simulink model "sampleModel7126_pp_difftest"  (R2018a)
settings: Solver=VariableStepAuto  StartTime=0.0  StopTime=10.0  RelTol=1e-3
undefined symbols (not defined in the file or in its folder): DiscIntNeverNeededParam
libraries: simulink x367
(part 5 of 8)

== system sampleModel7126_pp_difftest/cfblk293 ==
  cfblk1 : Inport
  cfblk9 : Inport  Port=2
  Action Port : ActionPort  ActionType=then
  cfblk{6,10..13} (5 alike) : Delay
  cfblk3 : simulink/Continuous/PID Controller (2DOF)  Controller=PID  TimeDomain=Discrete-time  SampleTime=-1  IntegratorMethod=Forward Euler  FilterMethod=Forward Euler  Form=Parallel  UseFilter=on  ControllerParametersSource=internal  P=1  I=1  D=0  N=100  b=1  c=1  InitialConditionSource=internal  InitialConditionForIntegrator=0  InitialConditionForFilter=0  ExternalReset=none  LimitOutput=off  UpperSaturationLimit=inf  LowerSaturationLimit=-inf  LinearizeAsGain=off  AntiWindupMode=none  Kb=1  TrackingMode=off  Kt=1  PParamMin=[]  PParamMax=[]  IParamMin=[]  IParamMax=[]  DParamMin=[]  DParamMax=[]  NParamMin=[]  NParamMax=[]  bParamMin=[]  bParamMax=[]  cParamMin=[]  cParamMax=[]  KbParamMin=[]  KbParamMax=[]  KtParamMin=[]  KtParamMax=[]  POutMin=[]  POutMax=[]  IOutMin=[]  IOutMax=[]  DOutMin=[]  DOutMax=[]  NOutMin=[]  NOutMax=[]  bOutMin=[]  bOutMax=[]  cOutMin=[]  cOutMax=[]  KbOutMin=[]  KbOutMax=[]  KtOutMin=[]  KtOutMax=[]  IntegratorOutMin=[]  IntegratorOutMax=[]  FilterOutMin=[]  FilterOutMax=[]  SumOutMin=[]  SumOutMax=[]  Sum1OutMin=[]  Sum1OutMax=[]  Sum2OutMin=[]  Sum2OutMax=[]  Sum3OutMin=[]  Sum3OutMax=[]  SumI1OutMin=[]  SumI1OutMax=[]  SumI2OutMin=[]  SumI2OutMax=[]  SumI3OutMin=[]  SumI3OutMax=[]  SumDOutMin=[]  SumDOutMax=[]  SaturationOutMin=[]  SaturationOutMax=[]  IntegratorContinuousStateAttributes=''  IntegratorStateMustResolveToSignalObject=off  IntegratorRTWStateStorageClass=Auto  FilterContinuousStateAttributes=''  FilterStateMustResolveToSignalObject=off  FilterRTWStateStorageClass=Auto  DifferentiatorICPrevScaledInput=0  DifferentiatorOutMin=[]  DifferentiatorOutMax=[]  FilterDiffOutCoefMin=[]  FilterDiffOutCoefMax=[]  SumDenOutMin=[]  SumDenOutMax=[]  SumNumOutMin=[]  SumNumOutMax=[]  ReciprocalOutMin=[]  ReciprocalOutMax=[]  DivideOutMin=[]  DivideOutMax=[]  TunerSelectOption=Transfer Function Based (PID Tuner App)
  cfblk4 : Delay  ShowEnablePort=on
      settings: InputPortMap=u0,e6
  cfblk5 : Delay  ShowEnablePort=on
      settings: InputPortMap=u0,e6
  cfblk7 : simulink/Continuous/PID Controller (2DOF)  Controller=PID  TimeDomain=Discrete-time  SampleTime=-1  IntegratorMethod=Forward Euler  FilterMethod=Forward Euler  Form=Parallel  UseFilter=on  ControllerParametersSource=internal  P=1  I=1  D=0  N=100  b=1  c=1  InitialConditionSource=internal  InitialConditionForIntegrator=0  InitialConditionForFilter=0  ExternalReset=none  LimitOutput=off  UpperSaturationLimit=inf  LowerSaturationLimit=-inf  LinearizeAsGain=off  AntiWindupMode=none  Kb=1  TrackingMode=off  Kt=1  PParamMin=[]  PParamMax=[]  IParamMin=[]  IParamMax=[]  DParamMin=[]  DParamMax=[]  NParamMin=[]  NParamMax=[]  bParamMin=[]  bParamMax=[]  cParamMin=[]  cParamMax=[]  KbParamMin=[]  KbParamMax=[]  KtParamMin=[]  KtParamMax=[]  POutMin=[]  POutMax=[]  IOutMin=[]  IOutMax=[]  DOutMin=[]  DOutMax=[]  NOutMin=[]  NOutMax=[]  bOutMin=[]  bOutMax=[]  cOutMin=[]  cOutMax=[]  KbOutMin=[]  KbOutMax=[]  KtOutMin=[]  KtOutMax=[]  IntegratorOutMin=[]  IntegratorOutMax=[]  FilterOutMin=[]  FilterOutMax=[]  SumOutMin=[]  SumOutMax=[]  Sum1OutMin=[]  Sum1OutMax=[]  Sum2OutMin=[]  Sum2OutMax=[]  Sum3OutMin=[]  Sum3OutMax=[]  SumI1OutMin=[]  SumI1OutMax=[]  SumI2OutMin=[]  SumI2OutMax=[]  SumI3OutMin=[]  SumI3OutMax=[]  SumDOutMin=[]  SumDOutMax=[]  SaturationOutMin=[]  SaturationOutMax=[]  IntegratorContinuousStateAttributes=''  IntegratorStateMustResolveToSignalObject=off  IntegratorRTWStateStorageClass=Auto  FilterContinuousStateAttributes=''  FilterStateMustResolveToSignalObject=off  FilterRTWStateStorageClass=Auto  DifferentiatorICPrevScaledInput=0  DifferentiatorOutMin=[]  DifferentiatorOutMax=[]  FilterDiffOutCoefMin=[]  FilterDiffOutCoefMax=[]  SumDenOutMin=[]  SumDenOutMax=[]  SumNumOutMin=[]  SumNumOutMax=[]  ReciprocalOutMin=[]  ReciprocalOutMax=[]  DivideOutMin=[]  DivideOutMax=[]  TunerSelectOption=Transfer Function Based (PID Tuner App)
  cfblk8 : simulink/Discrete/Transfer Fcn First Order  PoleZ=0.95  ICPrevOutput=0.0  DoSatur=off
      settings: SourceProductName=Simulink
  cyemi_{1188..1201} (14 alike) : DataTypeConversion  OutDataTypeStr=double
  cfblk2 : Outport
  wires:
  cfblk7/1 -> cyemi_1189/1, cyemi_1190/1, cyemi_1191/1
  cfblk1/1 -> cfblk2/1
  cfblk8/1 -> cyemi_1188/1, cyemi_1200/1
  cyemi_1188/1 -> cfblk10/1
  cyemi_1189/1 -> cfblk11/1
  cyemi_1190/1 -> cfblk12/1
  cyemi_1191/1 -> cfblk13/1
  cyemi_1192/1 -> cfblk3/1
  cfblk10/1 -> cyemi_1192/1
  cyemi_1193/1 -> cfblk3/2
  cfblk13/1 -> cyemi_1193/1
  cyemi_1194/1 -> cfblk4/1
  cfblk5/1 -> cyemi_1194/1
  cyemi_1195/1 -> cfblk4/2
  cfblk12/1 -> cyemi_1195/1
  cyemi_1196/1 -> cfblk5/1
  cfblk11/1 -> cyemi_1196/1
  cyemi_1197/1 -> cfblk5/2
  cfblk3/1 -> cyemi_1197/1
  cyemi_1198/1 -> cfblk6/1
  cfblk4/1 -> cyemi_1198/1
  cyemi_1199/1 -> cfblk7/1
  cfblk9/1 -> cyemi_1199/1
  cyemi_1200/1 -> cfblk7/2
  cyemi_1201/1 -> cfblk8/1
  cfblk6/1 -> cyemi_1201/1

== system sampleModel7126_pp_difftest/cfblk294 ==
  cfblk1 : Inport
  cfblk9 : Inport  Port=2
  cfblk10 : Inport  Port=3
  Action Port : ActionPort  ActionType=else
  cfblk11 : Delay
  cfblk12 : Delay
  cfblk3 : Delay  DelayLengthSource=Input port
      settings: InputPortMap=u0,p1
  cfblk4 : Delay  DelayLengthSource=Input port
      settings: InputPortMap=u0,p1
  cfblk5 : simulink/Discrete/Tapped Delay  vinit=0.0  samptime=-1  NumDelays=1  DelayOrder=Oldest  includeCurrent=off
  cfblk6 : Delay  DelayLengthSource=Input port
      settings: InputPortMap=u0,p1
  cfblk7 : Delay
  cfblk8 : simulink/Discrete/Transfer Fcn First Order  PoleZ=0.95  ICPrevOutput=0.0  DoSatur=off
      settings: SourceProductName=Simulink
  cyemi_{1205..1215} (11 alike) : DataTypeConversion  OutDataTypeStr=double
  cfblk2 : Outport
  wires:
  cfblk9/1 -> cfblk2/1
  cfblk7/1 -> cyemi_1209/1, cyemi_1211/1
  cyemi_1205/1 -> cfblk11/1
  cfblk8/1 -> cyemi_1205/1
  cyemi_1206/1 -> cfblk12/1
  cfblk6/1 -> cyemi_1206/1
  cyemi_1207/1 -> cfblk3/1
  cfblk11/1 -> cyemi_1207/1
  cyemi_1208/1 -> cfblk3/2
  cfblk1/1 -> cyemi_1208/1
  cyemi_1209/1 -> cfblk4/1
  cyemi_1210/1 -> cfblk4/2
  cfblk12/1 -> cyemi_1210/1
  cyemi_1211/1 -> cfblk5/1
  cyemi_1212/1 -> cfblk6/1
  cfblk5/1 -> cyemi_1212/1
  cyemi_1213/1 -> cfblk6/2
  cfblk4/1 -> cyemi_1213/1
  cyemi_1214/1 -> cfblk7/1
  cfblk10/1 -> cyemi_1214/1
  cyemi_1215/1 -> cfblk8/1
  cfblk3/1 -> cyemi_1215/1

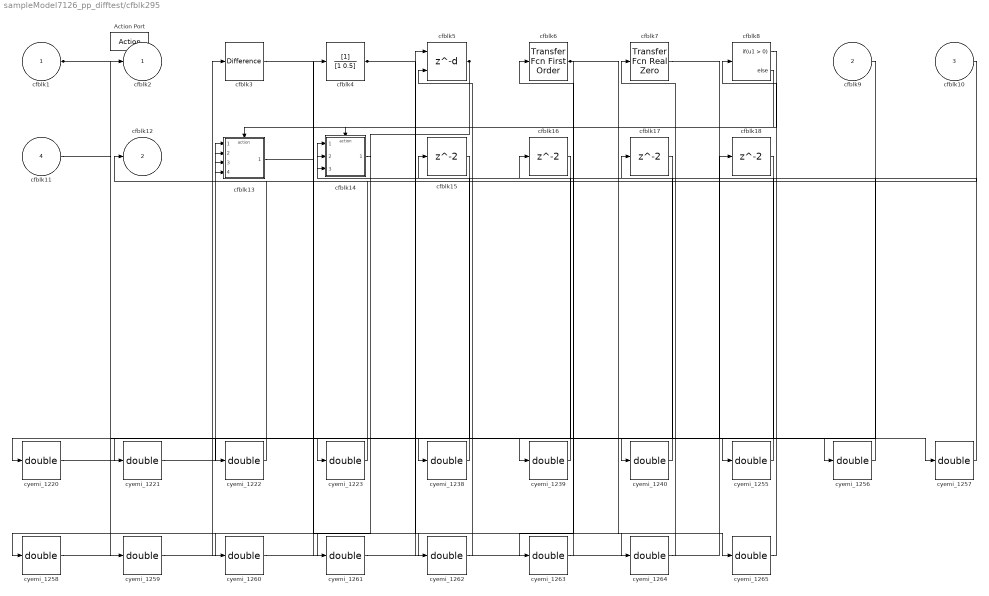
== system sampleModel7126_pp_difftest/cfblk295 ==
  cfblk1 : Inport
  cfblk9 : Inport  Port=2
  cfblk10 : Inport  Port=3
  cfblk11 : Inport  Port=4
  Action Port : ActionPort  ActionType=then
  cfblk13 : Subsystem  TreatAsAtomicUnit=on
  cfblk14 : Subsystem  TreatAsAtomicUnit=on
  cfblk{15..18} (4 alike) : Delay
  cfblk3 : simulink/Discrete/Difference  ICPrevInput=0.0  OutMin=[]  OutMax=[]  OutDataTypeStr=double  OutputDataTypeScalingMode=double  OutDataType=fixdt(1, 16)  OutScaling=2^-10  DoSatur=off
  cfblk4 : DiscreteFilter
  cfblk5 : Delay  DelayLengthSource=Input port
      settings: InputPortMap=u0,p1
  cfblk6 : simulink/Discrete/Transfer Fcn First Order  PoleZ=0.95  ICPrevOutput=0.0  DoSatur=off
      settings: SourceProductName=Simulink
  cfblk7 : simulink/Discrete/Transfer Fcn Real Zero  ZeroZ=0.75  ICPrevInput=0.0  DoSatur=off
      settings: SourceProductName=Simulink  SourceProductBaseCode=SL
  cfblk8 : If  SampleTime=1
  cyemi_{1220..1223,1238..1240,1255..1265} (18 alike) : DataTypeConversion  OutDataTypeStr=double
  cfblk2 : Outport
  cfblk12 : Outport  Port=2
  wires:
  cfblk4/1 -> cyemi_1255/1, cyemi_1264/1
  cfblk5/1 -> cyemi_1258/1, cyemi_1260/1
  cfblk10/1 -> cfblk12/1
  cfblk1/1 -> cfblk2/1, cyemi_1223/1, cyemi_1240/1
  cfblk6/1 -> cyemi_1239/1, cyemi_1265/1
  cfblk8/1 -> cfblk13/Action
  cfblk8/2 -> cfblk14/Action
  cyemi_1220/1 -> cfblk13/1(cfblk1)
  cfblk15/1 -> cyemi_1220/1
  cyemi_1221/1 -> cfblk13/2(cfblk15)
  cfblk17/1 -> cyemi_1221/1
  cyemi_1222/1 -> cfblk13/3(cfblk16)
  cfblk18/1 -> cyemi_1222/1
  cyemi_1223/1 -> cfblk13/4(cfblk17)
  cyemi_1238/1 -> cfblk14/1(cfblk1)
  cfblk16/1 -> cyemi_1238/1
  cyemi_1239/1 -> cfblk14/2(cfblk14)
  cyemi_1240/1 -> cfblk14/3(cfblk15)
  cyemi_1255/1 -> cfblk15/1
  cyemi_1256/1 -> cfblk16/1
  cfblk13/1(cfblk2) -> cyemi_1256/1
  cyemi_1257/1 -> cfblk17/1
  cfblk7/1 -> cyemi_1257/1
  cyemi_1258/1 -> cfblk18/1
  cyemi_1259/1 -> cfblk3/1
  cfblk11/1 -> cyemi_1259/1
  cyemi_1260/1 -> cfblk4/1
  cyemi_1261/1 -> cfblk5/1
  cfblk14/1(cfblk2) -> cyemi_1261/1
  cyemi_1262/1 -> cfblk5/2
  cfblk3/1 -> cyemi_1262/1
  cyemi_1263/1 -> cfblk6/1
  cfblk9/1 -> cyemi_1263/1
  cyemi_1264/1 -> cfblk7/1
  cyemi_1265/1 -> cfblk8/1

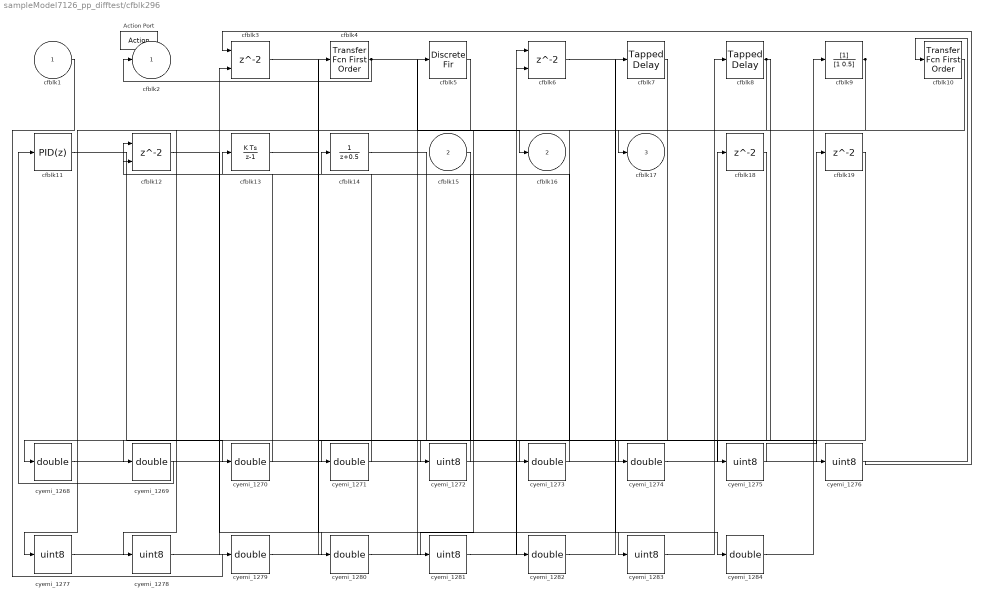
== system sampleModel7126_pp_difftest/cfblk296 ==
  cfblk1 : Inport
  cfblk15 : Inport  Port=2
  Action Port : ActionPort  ActionType=else
  cfblk10 : simulink/Discrete/Transfer Fcn First Order  PoleZ=0.95  ICPrevOutput=0.0  DoSatur=off
      settings: SourceProductName=Simulink
  cfblk11 : simulink/Continuous/PID Controller  Controller=PID  TimeDomain=Discrete-time  SampleTime=-1  IntegratorMethod=Forward Euler  FilterMethod=Forward Euler  Form=Parallel  UseFilter=on  ControllerParametersSource=internal  P=1  I=1  D=0  N=100  InitialConditionSource=internal  InitialConditionForIntegrator=0  InitialConditionForFilter=0  ExternalReset=none  LimitOutput=off  UpperSaturationLimit=inf  LowerSaturationLimit=-inf  LinearizeAsGain=off  AntiWindupMode=none  Kb=1  TrackingMode=off  Kt=1  PParamMin=[]  PParamMax=[]  IParamMin=[]  IParamMax=[]  DParamMin=[]  DParamMax=[]  NParamMin=[]  NParamMax=[]  KbParamMin=[]  KbParamMax=[]  KtParamMin=[]  KtParamMax=[]  POutMin=[]  POutMax=[]  IOutMin=[]  IOutMax=[]  DOutMin=[]  DOutMax=[]  NOutMin=[]  NOutMax=[]  KbOutMin=[]  KbOutMax=[]  KtOutMin=[]  KtOutMax=[]  IntegratorOutMin=[]  IntegratorOutMax=[]  FilterOutMin=[]  FilterOutMax=[]  SumOutMin=[]  SumOutMax=[]  SumI1OutMin=[]  SumI1OutMax=[]  SumI2OutMin=[]  SumI2OutMax=[]  SumI3OutMin=[]  SumI3OutMax=[]  SumDOutMin=[]  SumDOutMax=[]  SaturationOutMin=[]  SaturationOutMax=[]  IntegratorContinuousStateAttributes=''  IntegratorStateMustResolveToSignalObject=off  IntegratorRTWStateStorageClass=Auto  FilterContinuousStateAttributes=''  FilterStateMustResolveToSignalObject=off  FilterRTWStateStorageClass=Auto  DifferentiatorICPrevScaledInput=0  DifferentiatorOutMin=[]  DifferentiatorOutMax=[]  FilterDiffOutCoefMin=[]  FilterDiffOutCoefMax=[]  SumDenOutMin=[]  SumDenOutMax=[]  SumNumOutMin=[]  SumNumOutMax=[]  ReciprocalOutMin=[]  ReciprocalOutMax=[]  DivideOutMin=[]  DivideOutMax=[]  TunerSelectOption=Transfer Function Based (PID Tuner App)
  cfblk12 : Delay  ShowEnablePort=on
      settings: InputPortMap=u0,e6
  cfblk13 : DiscreteIntegrator  SampleTime=-1  OutDataTypeStr=uint8  ICPrevOutput=DiscIntNeverNeededParam  ICPrevScaledInput=DiscIntNeverNeededParam
  cfblk14 : DiscreteTransferFcn
  cfblk18 : Delay
  cfblk19 : Delay
  cfblk3 : Delay  ShowEnablePort=on
      settings: InputPortMap=u0,e6
  cfblk4 : simulink/Discrete/Transfer Fcn First Order  PoleZ=0.95  ICPrevOutput=0.0  DoSatur=off
      settings: SourceProductName=Simulink
  cfblk5 : DiscreteFir
  cfblk6 : Delay  ShowEnablePort=on
      settings: InputPortMap=u0,e6
  cfblk7 : simulink/Discrete/Tapped Delay  vinit=0.0  samptime=-1  NumDelays=1  DelayOrder=Oldest  includeCurrent=off
  cfblk8 : simulink/Discrete/Tapped Delay  vinit=0.0  samptime=-1  NumDelays=1  DelayOrder=Oldest  includeCurrent=off
  cfblk9 : DiscreteFilter
  cyemi_{1268..1271,1273..1274,1279..1280,1282,1284} (10 alike) : DataTypeConversion  OutDataTypeStr=double
  cyemi_{1272,1275..1278,1281,1283} (7 alike) : DataTypeConversion  OutDataTypeStr=uint8
  cfblk2 : Outport
  cfblk16 : Outport  Port=2
  cfblk17 : Outport  Port=3
  wires:
  cfblk10/1 -> cfblk17/1
  cfblk4/1 -> cfblk2/1, cfblk16/1
  cfblk8/1 -> cyemi_1275/1, cyemi_1278/1, cyemi_1281/1
  cfblk9/1 -> cyemi_1268/1, cyemi_1273/1
  cyemi_1268/1 -> cfblk10/1
  cyemi_1269/1 -> cfblk11/1
  cfblk5/1 -> cyemi_1269/1
  cyemi_1270/1 -> cfblk12/1
  cfblk11/1 -> cyemi_1270/1
  cyemi_1271/1 -> cfblk12/2
  cfblk18/1 -> cyemi_1271/1
  cyemi_1272/1 -> cfblk13/1
  cfblk15/1 -> cyemi_1272/1
  cyemi_1273/1 -> cfblk14/1
  cyemi_1274/1 -> cfblk18/1
  cfblk7/1 -> cyemi_1274/1
  cyemi_1275/1 -> cfblk19/1
  cyemi_1276/1 -> cfblk3/1
  cfblk13/1 -> cyemi_1276/1
  cyemi_1277/1 -> cfblk3/2
  cfblk19/1 -> cyemi_1277/1
  cyemi_1278/1 -> cfblk4/1
  cyemi_1279/1 -> cfblk5/1
  cfblk1/1 -> cyemi_1279/1
  cyemi_1280/1 -> cfblk6/1
  cfblk12/1 -> cyemi_1280/1
  cyemi_1281/1 -> cfblk6/2
  cyemi_1282/1 -> cfblk7/1
  cfblk14/1 -> cyemi_1282/1
  cyemi_1283/1 -> cfblk8/1
  cfblk3/1 -> cyemi_1283/1
  cyemi_1284/1 -> cfblk9/1
  cfblk6/1 -> cyemi_1284/1

== system sampleModel7126_pp_difftest/cfblk297 ==
  cfblk1 : Inport
  cfblk8 : Inport  Port=2
  cfblk9 : Inport  Port=3
  Action Port : ActionPort  ActionType=then
  cfblk11 : Delay
  cfblk3 : DiscreteFilter
  cfblk4 : simulink/Discrete/Tapped Delay  vinit=0.0  samptime=-1  NumDelays=1  DelayOrder=Oldest  includeCurrent=off
  cfblk5 : simulink/Continuous/PID Controller  Controller=PID  TimeDomain=Discrete-time  SampleTime=-1  IntegratorMethod=Forward Euler  FilterMethod=Forward Euler  Form=Parallel  UseFilter=on  ControllerParametersSource=internal  P=1  I=1  D=0  N=100  InitialConditionSource=internal  InitialConditionForIntegrator=0  InitialConditionForFilter=0  ExternalReset=none  LimitOutput=off  UpperSaturationLimit=inf  LowerSaturationLimit=-inf  LinearizeAsGain=off  AntiWindupMode=none  Kb=1  TrackingMode=off  Kt=1  PParamMin=[]  PParamMax=[]  IParamMin=[]  IParamMax=[]  DParamMin=[]  DParamMax=[]  NParamMin=[]  NParamMax=[]  KbParamMin=[]  KbParamMax=[]  KtParamMin=[]  KtParamMax=[]  POutMin=[]  POutMax=[]  IOutMin=[]  IOutMax=[]  DOutMin=[]  DOutMax=[]  NOutMin=[]  NOutMax=[]  KbOutMin=[]  KbOutMax=[]  KtOutMin=[]  KtOutMax=[]  IntegratorOutMin=[]  IntegratorOutMax=[]  FilterOutMin=[]  FilterOutMax=[]  SumOutMin=[]  SumOutMax=[]  SumI1OutMin=[]  SumI1OutMax=[]  SumI2OutMin=[]  SumI2OutMax=[]  SumI3OutMin=[]  SumI3OutMax=[]  SumDOutMin=[]  SumDOutMax=[]  SaturationOutMin=[]  SaturationOutMax=[]  IntegratorContinuousStateAttributes=''  IntegratorStateMustResolveToSignalObject=off  IntegratorRTWStateStorageClass=Auto  FilterContinuousStateAttributes=''  FilterStateMustResolveToSignalObject=off  FilterRTWStateStorageClass=Auto  DifferentiatorICPrevScaledInput=0  DifferentiatorOutMin=[]  DifferentiatorOutMax=[]  FilterDiffOutCoefMin=[]  FilterDiffOutCoefMax=[]  SumDenOutMin=[]  SumDenOutMax=[]  SumNumOutMin=[]  SumNumOutMax=[]  ReciprocalOutMin=[]  ReciprocalOutMax=[]  DivideOutMin=[]  DivideOutMax=[]  TunerSelectOption=Transfer Function Based (PID Tuner App)
  cfblk6 : simulink/Discrete/Difference  ICPrevInput=0.0  OutMin=[]  OutMax=[]  OutDataTypeStr=double  OutputDataTypeScalingMode=double  OutDataType=fixdt(1, 16)  OutScaling=2^-10  DoSatur=off
  cfblk7 : simulink/Continuous/PID Controller (2DOF)  Controller=PID  TimeDomain=Discrete-time  SampleTime=-1  IntegratorMethod=Forward Euler  FilterMethod=Forward Euler  Form=Parallel  UseFilter=on  ControllerParametersSource=internal  P=1  I=1  D=0  N=100  b=1  c=1  InitialConditionSource=internal  InitialConditionForIntegrator=0  InitialConditionForFilter=0  ExternalReset=none  LimitOutput=off  UpperSaturationLimit=inf  LowerSaturationLimit=-inf  LinearizeAsGain=off  AntiWindupMode=none  Kb=1  TrackingMode=off  Kt=1  PParamMin=[]  PParamMax=[]  IParamMin=[]  IParamMax=[]  DParamMin=[]  DParamMax=[]  NParamMin=[]  NParamMax=[]  bParamMin=[]  bParamMax=[]  cParamMin=[]  cParamMax=[]  KbParamMin=[]  KbParamMax=[]  KtParamMin=[]  KtParamMax=[]  POutMin=[]  POutMax=[]  IOutMin=[]  IOutMax=[]  DOutMin=[]  DOutMax=[]  NOutMin=[]  NOutMax=[]  bOutMin=[]  bOutMax=[]  cOutMin=[]  cOutMax=[]  KbOutMin=[]  KbOutMax=[]  KtOutMin=[]  KtOutMax=[]  IntegratorOutMin=[]  IntegratorOutMax=[]  FilterOutMin=[]  FilterOutMax=[]  SumOutMin=[]  SumOutMax=[]  Sum1OutMin=[]  Sum1OutMax=[]  Sum2OutMin=[]  Sum2OutMax=[]  Sum3OutMin=[]  Sum3OutMax=[]  SumI1OutMin=[]  SumI1OutMax=[]  SumI2OutMin=[]  SumI2OutMax=[]  SumI3OutMin=[]  SumI3OutMax=[]  SumDOutMin=[]  SumDOutMax=[]  SaturationOutMin=[]  SaturationOutMax=[]  IntegratorContinuousStateAttributes=''  IntegratorStateMustResolveToSignalObject=off  IntegratorRTWStateStorageClass=Auto  FilterContinuousStateAttributes=''  FilterStateMustResolveToSignalObject=off  FilterRTWStateStorageClass=Auto  DifferentiatorICPrevScaledInput=0  DifferentiatorOutMin=[]  DifferentiatorOutMax=[]  FilterDiffOutCoefMin=[]  FilterDiffOutCoefMax=[]  SumDenOutMin=[]  SumDenOutMax=[]  SumNumOutMin=[]  SumNumOutMax=[]  ReciprocalOutMin=[]  ReciprocalOutMax=[]  DivideOutMin=[]  DivideOutMax=[]  TunerSelectOption=Transfer Function Based (PID Tuner App)
  cyemi_{1288..1294} (7 alike) : DataTypeConversion  OutDataTypeStr=double
  cfblk2 : Outport
  cfblk10 : Outport  Port=2
  wires:
  cfblk1/1 -> cfblk10/1
  cfblk6/1 -> cfblk2/1
  cyemi_1288/1 -> cfblk11/1
  cfblk7/1 -> cyemi_1288/1
  cyemi_1289/1 -> cfblk3/1
  cfblk11/1 -> cyemi_1289/1
  cyemi_1290/1 -> cfblk4/1
  cfblk9/1 -> cyemi_1290/1
  cyemi_1291/1 -> cfblk5/1
  cfblk8/1 -> cyemi_1291/1
  cyemi_1292/1 -> cfblk6/1
  cfblk4/1 -> cyemi_1292/1
  cyemi_1293/1 -> cfblk7/1
  cfblk5/1 -> cyemi_1293/1
  cyemi_1294/1 -> cfblk7/2
  cfblk3/1 -> cyemi_1294/1

== system sampleModel7126_pp_difftest/cfblk298 ==
  cfblk1 : Inport
  cfblk9 : Inport  Port=2
  cfblk10 : Inport  Port=3
  cfblk11 : Inport  Port=4
  Action Port : ActionPort  ActionType=else
  cfblk15 : Subsystem  TreatAsAtomicUnit=on
  cfblk16 : Subsystem  TreatAsAtomicUnit=on
  cfblk{3..4,17..19} (5 alike) : Delay
  cfblk5 : DiscreteZeroPole  Poles=[0 0.5]  Gain=1  SampleTime=-1
  cfblk6 : DiscreteZeroPole  Poles=[0 0.5]  Gain=1  SampleTime=-1
  cfblk7 : DiscreteFilter
  cfblk8 : If  SampleTime=1
  cyemi_{1299..1300,1314,1331..1339} (12 alike) : DataTypeConversion  OutDataTypeStr=double
  cfblk2 : Outport
  cfblk12 : Outport  Port=2
  cfblk13 : Outport  Port=3
  cfblk14 : Outport  Port=4
  wires:
  cfblk10/1 -> cfblk14/1
  cfblk4/1 -> cfblk2/1
  cfblk15/1(cfblk2) -> cfblk12/1
  cfblk9/1 -> cfblk13/1
  cfblk8/1 -> cfblk15/Action
  cfblk8/2 -> cfblk16/Action
  cyemi_1299/1 -> cfblk15/1(cfblk1)
  cfblk11/1 -> cyemi_1299/1, cyemi_1300/1
  cyemi_1300/1 -> cfblk15/2(cfblk14)
  cyemi_1314/1 -> cfblk16/1(cfblk1)
  cfblk7/1 -> cyemi_1314/1
  cyemi_1331/1 -> cfblk17/1
  cfblk6/1 -> cyemi_1331/1
  cyemi_1332/1 -> cfblk18/1
  cfblk16/1(cfblk2) -> cyemi_1332/1
  cyemi_1333/1 -> cfblk19/1
  cfblk15/2(cfblk15) -> cyemi_1333/1
  cyemi_1334/1 -> cfblk3/1
  cfblk17/1 -> cyemi_1334/1
  cyemi_1335/1 -> cfblk4/1
  cfblk1/1 -> cyemi_1335/1
  cyemi_1336/1 -> cfblk5/1
  cfblk18/1 -> cyemi_1336/1
  cyemi_1337/1 -> cfblk6/1
  cfblk3/1 -> cyemi_1337/1
  cyemi_1338/1 -> cfblk7/1
  cfblk5/1 -> cyemi_1338/1
  cyemi_1339/1 -> cfblk8/1
  cfblk19/1 -> cyemi_1339/1

== system sampleModel7126_pp_difftest/cfblk245/cfblk18 ==
  cfblk1 : Inport
  cfblk9 : Inport  Port=2
  Action Port : ActionPort  ActionType=then
  cfblk3 : UnitDelay  SampleTime=-1
  cfblk4 : Delay  ShowEnablePort=on
      settings: InputPortMap=u0,e6
  cfblk5 : DiscreteFilter
  cfblk6 : simulink/Discrete/Transfer Fcn Real Zero  ZeroZ=0.75  ICPrevInput=0.0  DoSatur=off
      settings: SourceProductName=Simulink  SourceProductBaseCode=SL
  cfblk7 : simulink/Discrete/Transfer Fcn Lead or Lag  PoleZ=0.95  ZeroZ=0.75  ICPrevOutput=0.0  ICPrevInput=0.0  DoSatur=off
      settings: SourceProductName=Simulink  SourceProductBaseCode=SL
  cfblk8 : Delay  DelayLengthSource=Input port
      settings: InputPortMap=u0,p1
  cyemi_{71..78} (8 alike) : DataTypeConversion  OutDataTypeStr=double
  cfblk2 : Outport
  cfblk10 : Outport  Port=2
  cfblk11 : Outport  Port=3
  wires:
  cfblk5/1 -> cfblk11/1
  cfblk3/1 -> cfblk10/1, cyemi_73/1, cyemi_74/1
  cfblk8/1 -> cfblk2/1
  cyemi_71/1 -> cfblk3/1
  cfblk7/1 -> cyemi_71/1
  cyemi_72/1 -> cfblk4/1
  cfblk6/1 -> cyemi_72/1
  cyemi_73/1 -> cfblk4/2
  cyemi_74/1 -> cfblk5/1
  cyemi_75/1 -> cfblk6/1
  cfblk9/1 -> cyemi_75/1
  cyemi_76/1 -> cfblk7/1
  cfblk1/1 -> cyemi_76/1
  cyemi_77/1 -> cfblk8/1
  cfblk4/1 -> cyemi_77/1, cyemi_78/1
  cyemi_78/1 -> cfblk8/2

== system sampleModel7126_pp_difftest/cfblk245/cfblk19 ==
  cfblk1 : Inport
  Action Port : ActionPort  ActionType=else
  cfblk10 : DiscreteZeroPole  Poles=[0 0.5]  Gain=1  SampleTime=-1
  cfblk13 : Delay
  cfblk3 : DiscreteStateSpace  SampleTime=-1
  cfblk4 : DiscreteZeroPole  Poles=[0 0.5]  Gain=1  SampleTime=-1
  cfblk5 : DiscreteZeroPole  Poles=[0 0.5]  Gain=1  SampleTime=-1
  cfblk6 : simulink/Discrete/Transfer Fcn First Order  PoleZ=0.95  ICPrevOutput=0.0  DoSatur=off
      settings: SourceProductName=Simulink
  cfblk7 : DiscreteFir
  cfblk8 : DiscreteIntegrator  SampleTime=-1  OutDataTypeStr=double  ICPrevOutput=DiscIntNeverNeededParam  ICPrevScaledInput=DiscIntNeverNeededParam
  cfblk9 : Delay  ShowEnablePort=on
      settings: InputPortMap=u0,e6
  cyemi_{80..89} (10 alike) : DataTypeConversion  OutDataTypeStr=double
  cfblk2 : Outport
  cfblk11 : Outport  Port=2
  cfblk12 : Outport  Port=3
  wires:
  cfblk8/1 -> cyemi_85/1, cyemi_88/1
  cfblk5/1 -> cfblk11/1, cyemi_87/1
  cfblk7/1 -> cfblk12/1
  cfblk1/1 -> cfblk2/1
  cfblk4/1 -> cyemi_80/1, cyemi_89/1
  cyemi_80/1 -> cfblk10/1
  cyemi_81/1 -> cfblk13/1
  cfblk6/1 -> cyemi_81/1
  cyemi_82/1 -> cfblk3/1
  cfblk9/1 -> cyemi_82/1
  cyemi_83/1 -> cfblk4/1
  cfblk13/1 -> cyemi_83/1
  cyemi_84/1 -> cfblk5/1
  cfblk10/1 -> cyemi_84/1
  cyemi_85/1 -> cfblk6/1
  cyemi_86/1 -> cfblk7/1
  cfblk3/1 -> cyemi_86/1
  cyemi_87/1 -> cfblk8/1
  cyemi_88/1 -> cfblk9/1
  cyemi_89/1 -> cfblk9/2

== system sampleModel7126_pp_difftest/cfblk246/cfblk10 ==
  cfblk1 : Inport
  cfblk13 : Inport  Port=2
  Action Port : ActionPort  ActionType=else
  cfblk10 : DiscreteStateSpace  SampleTime=-1
  cfblk11 : simulink/Discrete/Transfer Fcn Lead or Lag  PoleZ=0.95  ZeroZ=0.75  ICPrevOutput=0.0  ICPrevInput=0.0  DoSatur=off
      settings: SourceProductName=Simulink  SourceProductBaseCode=SL
  cfblk12 : simulink/Continuous/PID Controller (2DOF)  Controller=PID  TimeDomain=Discrete-time  SampleTime=-1  IntegratorMethod=Forward Euler  FilterMethod=Forward Euler  Form=Parallel  UseFilter=on  ControllerParametersSource=internal  P=1  I=1  D=0  N=100  b=1  c=1  InitialConditionSource=internal  InitialConditionForIntegrator=0  InitialConditionForFilter=0  ExternalReset=none  LimitOutput=off  UpperSaturationLimit=inf  LowerSaturationLimit=-inf  LinearizeAsGain=off  AntiWindupMode=none  Kb=1  TrackingMode=off  Kt=1  PParamMin=[]  PParamMax=[]  IParamMin=[]  IParamMax=[]  DParamMin=[]  DParamMax=[]  NParamMin=[]  NParamMax=[]  bParamMin=[]  bParamMax=[]  cParamMin=[]  cParamMax=[]  KbParamMin=[]  KbParamMax=[]  KtParamMin=[]  KtParamMax=[]  POutMin=[]  POutMax=[]  IOutMin=[]  IOutMax=[]  DOutMin=[]  DOutMax=[]  NOutMin=[]  NOutMax=[]  bOutMin=[]  bOutMax=[]  cOutMin=[]  cOutMax=[]  KbOutMin=[]  KbOutMax=[]  KtOutMin=[]  KtOutMax=[]  IntegratorOutMin=[]  IntegratorOutMax=[]  FilterOutMin=[]  FilterOutMax=[]  SumOutMin=[]  SumOutMax=[]  Sum1OutMin=[]  Sum1OutMax=[]  Sum2OutMin=[]  Sum2OutMax=[]  Sum3OutMin=[]  Sum3OutMax=[]  SumI1OutMin=[]  SumI1OutMax=[]  SumI2OutMin=[]  SumI2OutMax=[]  SumI3OutMin=[]  SumI3OutMax=[]  SumDOutMin=[]  SumDOutMax=[]  SaturationOutMin=[]  SaturationOutMax=[]  IntegratorContinuousStateAttributes=''  IntegratorStateMustResolveToSignalObject=off  IntegratorRTWStateStorageClass=Auto  FilterContinuousStateAttributes=''  FilterStateMustResolveToSignalObject=off  FilterRTWStateStorageClass=Auto  DifferentiatorICPrevScaledInput=0  DifferentiatorOutMin=[]  DifferentiatorOutMax=[]  FilterDiffOutCoefMin=[]  FilterDiffOutCoefMax=[]  SumDenOutMin=[]  SumDenOutMax=[]  SumNumOutMin=[]  SumNumOutMax=[]  ReciprocalOutMin=[]  ReciprocalOutMax=[]  DivideOutMin=[]  DivideOutMax=[]  TunerSelectOption=Transfer Function Based (PID Tuner App)
  cfblk16 : Delay
  cfblk17 : Delay
  cfblk3 : simulink/Discrete/Difference  ICPrevInput=0.0  OutMin=[]  OutMax=[]  OutDataTypeStr=double  OutputDataTypeScalingMode=double  OutDataType=fixdt(1, 16)  OutScaling=2^-10  DoSatur=off
  cfblk4 : DiscreteZeroPole  Poles=[0 0.5]  Gain=1  SampleTime=-1
  cfblk5 : Delay  DelayLengthSource=Input port
      settings: InputPortMap=u0,p1
  cfblk6 : Delay  DelayLengthSource=Input port
      settings: InputPortMap=u0,p1
  cfblk7 : simulink/Continuous/PID Controller  Controller=PID  TimeDomain=Discrete-time  SampleTime=-1  IntegratorMethod=Forward Euler  FilterMethod=Forward Euler  Form=Parallel  UseFilter=on  ControllerParametersSource=internal  P=1  I=1  D=0  N=100  InitialConditionSource=internal  InitialConditionForIntegrator=0  InitialConditionForFilter=0  ExternalReset=none  LimitOutput=off  UpperSaturationLimit=inf  LowerSaturationLimit=-inf  LinearizeAsGain=off  AntiWindupMode=none  Kb=1  TrackingMode=off  Kt=1  PParamMin=[]  PParamMax=[]  IParamMin=[]  IParamMax=[]  DParamMin=[]  DParamMax=[]  NParamMin=[]  NParamMax=[]  KbParamMin=[]  KbParamMax=[]  KtParamMin=[]  KtParamMax=[]  POutMin=[]  POutMax=[]  IOutMin=[]  IOutMax=[]  DOutMin=[]  DOutMax=[]  NOutMin=[]  NOutMax=[]  KbOutMin=[]  KbOutMax=[]  KtOutMin=[]  KtOutMax=[]  IntegratorOutMin=[]  IntegratorOutMax=[]  FilterOutMin=[]  FilterOutMax=[]  SumOutMin=[]  SumOutMax=[]  SumI1OutMin=[]  SumI1OutMax=[]  SumI2OutMin=[]  SumI2OutMax=[]  SumI3OutMin=[]  SumI3OutMax=[]  SumDOutMin=[]  SumDOutMax=[]  SaturationOutMin=[]  SaturationOutMax=[]  IntegratorContinuousStateAttributes=''  IntegratorStateMustResolveToSignalObject=off  IntegratorRTWStateStorageClass=Auto  FilterContinuousStateAttributes=''  FilterStateMustResolveToSignalObject=off  FilterRTWStateStorageClass=Auto  DifferentiatorICPrevScaledInput=0  DifferentiatorOutMin=[]  DifferentiatorOutMax=[]  FilterDiffOutCoefMin=[]  FilterDiffOutCoefMax=[]  SumDenOutMin=[]  SumDenOutMax=[]  SumNumOutMin=[]  SumNumOutMax=[]  ReciprocalOutMin=[]  ReciprocalOutMax=[]  DivideOutMin=[]  DivideOutMax=[]  TunerSelectOption=Transfer Function Based (PID Tuner App)
  cfblk8 : DiscreteZeroPole  Poles=[0 0.5]  Gain=1  SampleTime=-1
  cfblk9 : DiscreteFir
  cyemi_{103..117} (15 alike) : DataTypeConversion  OutDataTypeStr=double
  cfblk2 : Outport
  cfblk14 : Outport  Port=2
  cfblk15 : Outport  Port=3
  wires:
  cfblk9/1 -> cyemi_103/1, cyemi_108/1
  cfblk5/1 -> cfblk14/1, cfblk2/1
  cfblk6/1 -> cyemi_104/1, cyemi_112/1
  cfblk8/1 -> cfblk15/1, cyemi_114/1
  cyemi_103/1 -> cfblk10/1
  cyemi_104/1 -> cfblk11/1
  cyemi_105/1 -> cfblk12/1
  cfblk11/1 -> cyemi_105/1
  cyemi_106/1 -> cfblk12/2
  cfblk17/1 -> cyemi_106/1
  cyemi_107/1 -> cfblk16/1
  cfblk3/1 -> cyemi_107/1
  cyemi_108/1 -> cfblk17/1
  cyemi_109/1 -> cfblk3/1
  cfblk10/1 -> cyemi_109/1
  cyemi_110/1 -> cfblk4/1
  cfblk12/1 -> cyemi_110/1
  cyemi_111/1 -> cfblk5/1
  cfblk13/1 -> cyemi_111/1
  cyemi_112/1 -> cfblk5/2
  cyemi_113/1 -> cfblk6/1
  cfblk16/1 -> cyemi_113/1
  cyemi_114/1 -> cfblk6/2
  cyemi_115/1 -> cfblk7/1
  cfblk1/1 -> cyemi_115/1
  cyemi_116/1 -> cfblk8/1
  cfblk7/1 -> cyemi_116/1
  cyemi_117/1 -> cfblk9/1
  cfblk4/1 -> cyemi_117/1

== system sampleModel7126_pp_difftest/cfblk246/cfblk9 ==
  cfblk1 : Inport
  Action Port : ActionPort  ActionType=then
  cfblk10 : simulink/Discrete/Difference  ICPrevInput=0.0  OutMin=[]  OutMax=[]  OutDataTypeStr=double  OutputDataTypeScalingMode=double  OutDataType=fixdt(1, 16)  OutScaling=2^-10  DoSatur=off
  cfblk3 : Delay
  cfblk4 : simulink/Discrete/Tapped Delay  vinit=0.0  samptime=-1  NumDelays=1  DelayOrder=Oldest  includeCurrent=off
  cfblk5 : simulink/Discrete/Difference  ICPrevInput=0.0  OutMin=[]  OutMax=[]  OutDataTypeStr=double  OutputDataTypeScalingMode=double  OutDataType=fixdt(1, 16)  OutScaling=2^-10  DoSatur=off
  cfblk6 : simulink/Discrete/Transfer Fcn Lead or Lag  PoleZ=0.95  ZeroZ=0.75  ICPrevOutput=0.0  ICPrevInput=0.0  DoSatur=off
      settings: SourceProductName=Simulink  SourceProductBaseCode=SL
  cfblk7 : simulink/Discrete/Transfer Fcn Real Zero  ZeroZ=0.75  ICPrevInput=0.0  DoSatur=off
      settings: SourceProductName=Simulink  SourceProductBaseCode=SL
  cfblk8 : simulink/Discrete/Difference  ICPrevInput=0.0  OutMin=[]  OutMax=[]  OutDataTypeStr=double  OutputDataTypeScalingMode=double  OutDataType=fixdt(1, 16)  OutScaling=2^-10  DoSatur=off
  cfblk9 : UnitDelay  SampleTime=-1
  cyemi_{125..132} (8 alike) : DataTypeConversion  OutDataTypeStr=double
  cfblk2 : Outport
  cfblk11 : Outport  Port=2
  wires:
  cfblk8/1 -> cfblk2/1
  cfblk9/1 -> cyemi_125/1, cyemi_130/1
  cfblk3/1 -> cfblk11/1
  cyemi_125/1 -> cfblk10/1
  cyemi_126/1 -> cfblk3/1
  cfblk10/1 -> cyemi_126/1
  cyemi_127/1 -> cfblk4/1
  cfblk6/1 -> cyemi_127/1
  cyemi_128/1 -> cfblk5/1
  cfblk4/1 -> cyemi_128/1
  cyemi_129/1 -> cfblk6/1
  cfblk7/1 -> cyemi_129/1
  cyemi_130/1 -> cfblk7/1
  cyemi_131/1 -> cfblk8/1
  cfblk5/1 -> cyemi_131/1
  cyemi_132/1 -> cfblk9/1
  cfblk1/1 -> cyemi_132/1

== system sampleModel7126_pp_difftest/cfblk247/cfblk18 ==
  cfblk1 : Inport
  cfblk11 : Inport  Port=2
  cfblk12 : Inport  Port=3
  cfblk13 : Inport  Port=4
  Action Port : ActionPort  ActionType=then
  cfblk10 : DiscreteStateSpace  SampleTime=-1
  cfblk17 : Delay
  cfblk3 : DiscreteZeroPole  Poles=[0 0.5]  Gain=1  SampleTime=-1
  cfblk4 : DiscreteZeroPole  Poles=[0 0.5]  Gain=1  SampleTime=-1
  cfblk5 : simulink/Discrete/Difference  ICPrevInput=0.0  OutMin=[]  OutMax=[]  OutDataTypeStr=double  OutputDataTypeScalingMode=double  OutDataType=fixdt(1, 16)  OutScaling=2^-10  DoSatur=off
  cfblk6 : simulink/Discrete/Transfer Fcn Lead or Lag  PoleZ=0.95  ZeroZ=0.75  ICPrevOutput=0.0  ICPrevInput=0.0  DoSatur=off
      settings: SourceProductName=Simulink  SourceProductBaseCode=SL
  cfblk7 : DiscreteFilter
  cfblk8 : Delay  ShowEnablePort=on
      settings: InputPortMap=u0,e6
  cfblk9 : simulink/Discrete/Transfer Fcn Real Zero  ZeroZ=0.75  ICPrevInput=0.0  DoSatur=off
      settings: SourceProductName=Simulink  SourceProductBaseCode=SL
  cyemi_{145..154} (10 alike) : DataTypeConversion  OutDataTypeStr=double
  cfblk2 : Outport
  cfblk14 : Outport  Port=2
  cfblk15 : Outport  Port=3
  cfblk16 : Outport  Port=4
  wires:
  cfblk3/1 -> cfblk16/1
  cfblk13/1 -> cfblk14/1
  cfblk10/1 -> cfblk15/1
  cfblk6/1 -> cyemi_145/1, cyemi_149/1
  cfblk1/1 -> cfblk2/1
  cyemi_145/1 -> cfblk10/1
  cyemi_146/1 -> cfblk17/1
  cfblk7/1 -> cyemi_146/1
  cyemi_147/1 -> cfblk3/1
  cfblk11/1 -> cyemi_147/1
  cyemi_148/1 -> cfblk4/1
  cfblk5/1 -> cyemi_148/1
  cyemi_149/1 -> cfblk5/1
  cyemi_150/1 -> cfblk6/1
  cfblk12/1 -> cyemi_150/1
  cyemi_151/1 -> cfblk7/1
  cfblk9/1 -> cyemi_151/1
  cyemi_152/1 -> cfblk8/1
  cfblk17/1 -> cyemi_152/1
  cyemi_153/1 -> cfblk8/2
  cfblk4/1 -> cyemi_153/1
  cyemi_154/1 -> cfblk9/1
  cfblk8/1 -> cyemi_154/1

== system sampleModel7126_pp_difftest/cfblk247/cfblk19 ==
  cfblk1 : Inport
  cfblk11 : Inport  Port=2
  Action Port : ActionPort  ActionType=else
  cfblk10 : Delay
  cfblk14 : Delay
  cfblk3 : DiscreteFilter
  cfblk4 : simulink/Discrete/Tapped Delay  vinit=0.0  samptime=-1  NumDelays=1  DelayOrder=Oldest  includeCurrent=off
  cfblk5 : simulink/Discrete/Transfer Fcn First Order  PoleZ=0.95  ICPrevOutput=0.0  DoSatur=off
      settings: SourceProductName=Simulink
  cfblk6 : simulink/Discrete/Transfer Fcn Real Zero  ZeroZ=0.75  ICPrevInput=0.0  DoSatur=off
      settings: SourceProductName=Simulink  SourceProductBaseCode=SL
  cfblk7 : simulink/Continuous/PID Controller  Controller=PID  TimeDomain=Discrete-time  SampleTime=-1  IntegratorMethod=Forward Euler  FilterMethod=Forward Euler  Form=Parallel  UseFilter=on  ControllerParametersSource=internal  P=1  I=1  D=0  N=100  InitialConditionSource=internal  InitialConditionForIntegrator=0  InitialConditionForFilter=0  ExternalReset=none  LimitOutput=off  UpperSaturationLimit=inf  LowerSaturationLimit=-inf  LinearizeAsGain=off  AntiWindupMode=none  Kb=1  TrackingMode=off  Kt=1  PParamMin=[]  PParamMax=[]  IParamMin=[]  IParamMax=[]  DParamMin=[]  DParamMax=[]  NParamMin=[]  NParamMax=[]  KbParamMin=[]  KbParamMax=[]  KtParamMin=[]  KtParamMax=[]  POutMin=[]  POutMax=[]  IOutMin=[]  IOutMax=[]  DOutMin=[]  DOutMax=[]  NOutMin=[]  NOutMax=[]  KbOutMin=[]  KbOutMax=[]  KtOutMin=[]  KtOutMax=[]  IntegratorOutMin=[]  IntegratorOutMax=[]  FilterOutMin=[]  FilterOutMax=[]  SumOutMin=[]  SumOutMax=[]  SumI1OutMin=[]  SumI1OutMax=[]  SumI2OutMin=[]  SumI2OutMax=[]  SumI3OutMin=[]  SumI3OutMax=[]  SumDOutMin=[]  SumDOutMax=[]  SaturationOutMin=[]  SaturationOutMax=[]  IntegratorContinuousStateAttributes=''  IntegratorStateMustResolveToSignalObject=off  IntegratorRTWStateStorageClass=Auto  FilterContinuousStateAttributes=''  FilterStateMustResolveToSignalObject=off  FilterRTWStateStorageClass=Auto  DifferentiatorICPrevScaledInput=0  DifferentiatorOutMin=[]  DifferentiatorOutMax=[]  FilterDiffOutCoefMin=[]  FilterDiffOutCoefMax=[]  SumDenOutMin=[]  SumDenOutMax=[]  SumNumOutMin=[]  SumNumOutMax=[]  ReciprocalOutMin=[]  ReciprocalOutMax=[]  DivideOutMin=[]  DivideOutMax=[]  TunerSelectOption=Transfer Function Based (PID Tuner App)
  cfblk8 : UnitDelay  SampleTime=-1
  cfblk9 : simulink/Discrete/Transfer Fcn First Order  PoleZ=0.95  ICPrevOutput=0.0  DoSatur=off
      settings: SourceProductName=Simulink
  cyemi_{157..165} (9 alike) : DataTypeConversion  OutDataTypeStr=double
  cfblk2 : Outport
  cfblk12 : Outport  Port=2
  cfblk13 : Outport  Port=3
  wires:
  cfblk3/1 -> cfblk12/1
  cfblk7/1 -> cfblk2/1
  cfblk8/1 -> cfblk13/1
  cfblk11/1 -> cyemi_161/1, cyemi_164/1
  cyemi_157/1 -> cfblk10/1
  cfblk5/1 -> cyemi_157/1
  cyemi_158/1 -> cfblk14/1
  cfblk6/1 -> cyemi_158/1
  cyemi_159/1 -> cfblk3/1
  cfblk1/1 -> cyemi_159/1
  cyemi_160/1 -> cfblk4/1
  cfblk14/1 -> cyemi_160/1
  cyemi_161/1 -> cfblk5/1
  cyemi_162/1 -> cfblk6/1
  cfblk4/1 -> cyemi_162/1
  cyemi_163/1 -> cfblk7/1
  cfblk9/1 -> cyemi_163/1
  cyemi_164/1 -> cfblk8/1
  cyemi_165/1 -> cfblk9/1
  cfblk10/1 -> cyemi_165/1

== system sampleModel7126_pp_difftest/cfblk252/cfblk15 ==
  cfblk1 : Inport
  cfblk15 : Inport  Port=2
  Action Port : ActionPort  ActionType=then
  cfblk10 : DiscreteTransferFcn
  cfblk11 : simulink/Continuous/PID Controller (2DOF)  Controller=PID  TimeDomain=Discrete-time  SampleTime=-1  IntegratorMethod=Forward Euler  FilterMethod=Forward Euler  Form=Parallel  UseFilter=on  ControllerParametersSource=internal  P=1  I=1  D=0  N=100  b=1  c=1  InitialConditionSource=internal  InitialConditionForIntegrator=0  InitialConditionForFilter=0  ExternalReset=none  LimitOutput=off  UpperSaturationLimit=inf  LowerSaturationLimit=-inf  LinearizeAsGain=off  AntiWindupMode=none  Kb=1  TrackingMode=off  Kt=1  PParamMin=[]  PParamMax=[]  IParamMin=[]  IParamMax=[]  DParamMin=[]  DParamMax=[]  NParamMin=[]  NParamMax=[]  bParamMin=[]  bParamMax=[]  cParamMin=[]  cParamMax=[]  KbParamMin=[]  KbParamMax=[]  KtParamMin=[]  KtParamMax=[]  POutMin=[]  POutMax=[]  IOutMin=[]  IOutMax=[]  DOutMin=[]  DOutMax=[]  NOutMin=[]  NOutMax=[]  bOutMin=[]  bOutMax=[]  cOutMin=[]  cOutMax=[]  KbOutMin=[]  KbOutMax=[]  KtOutMin=[]  KtOutMax=[]  IntegratorOutMin=[]  IntegratorOutMax=[]  FilterOutMin=[]  FilterOutMax=[]  SumOutMin=[]  SumOutMax=[]  Sum1OutMin=[]  Sum1OutMax=[]  Sum2OutMin=[]  Sum2OutMax=[]  Sum3OutMin=[]  Sum3OutMax=[]  SumI1OutMin=[]  SumI1OutMax=[]  SumI2OutMin=[]  SumI2OutMax=[]  SumI3OutMin=[]  SumI3OutMax=[]  SumDOutMin=[]  SumDOutMax=[]  SaturationOutMin=[]  SaturationOutMax=[]  IntegratorContinuousStateAttributes=''  IntegratorStateMustResolveToSignalObject=off  IntegratorRTWStateStorageClass=Auto  FilterContinuousStateAttributes=''  FilterStateMustResolveToSignalObject=off  FilterRTWStateStorageClass=Auto  DifferentiatorICPrevScaledInput=0  DifferentiatorOutMin=[]  DifferentiatorOutMax=[]  FilterDiffOutCoefMin=[]  FilterDiffOutCoefMax=[]  SumDenOutMin=[]  SumDenOutMax=[]  SumNumOutMin=[]  SumNumOutMax=[]  ReciprocalOutMin=[]  ReciprocalOutMax=[]  DivideOutMin=[]  DivideOutMax=[]  TunerSelectOption=Transfer Function Based (PID Tuner App)
  cfblk12 : DiscreteZeroPole  Poles=[0 0.5]  Gain=1  SampleTime=-1
  cfblk13 : DiscreteFir
  cfblk14 : simulink/Discrete/Transfer Fcn Real Zero  ZeroZ=0.75  ICPrevInput=0.0  DoSatur=off
      settings: SourceProductName=Simulink  SourceProductBaseCode=SL
  cfblk17 : Delay
  cfblk18 : Delay
  cfblk3 : Delay
  cfblk4 : Delay  DelayLengthSource=Input port
      settings: InputPortMap=u0,p1
  cfblk5 : UnitDelay  SampleTime=-1
  cfblk6 : simulink/Discrete/Transfer Fcn Lead or Lag  PoleZ=0.95  ZeroZ=0.75  ICPrevOutput=0.0  ICPrevInput=0.0  DoSatur=off
      settings: SourceProductName=Simulink  SourceProductBaseCode=SL
  cfblk7 : DiscreteFilter
  cfblk8 : simulink/Discrete/Transfer Fcn Real Zero  ZeroZ=0.75  ICPrevInput=0.0  DoSatur=off
      settings: SourceProductName=Simulink  SourceProductBaseCode=SL
  cfblk9 : simulink/Discrete/Transfer Fcn Lead or Lag  PoleZ=0.95  ZeroZ=0.75  ICPrevOutput=0.0  ICPrevInput=0.0  DoSatur=off
      settings: SourceProductName=Simulink  SourceProductBaseCode=SL
  cyemi_{252..267} (16 alike) : DataTypeConversion  OutDataTypeStr=double
  cfblk2 : Outport
  cfblk16 : Outport  Port=2
  wires:
  cfblk3/1 -> cyemi_254/1, cyemi_255/1
  cfblk11/1 -> cyemi_258/1, cyemi_263/1
  cfblk12/1 -> cfblk16/1
  cfblk7/1 -> cfblk2/1
  cyemi_252/1 -> cfblk10/1
  cfblk9/1 -> cyemi_252/1
  cyemi_253/1 -> cfblk11/1
  cfblk13/1 -> cyemi_253/1
  cyemi_254/1 -> cfblk11/2
  cyemi_255/1 -> cfblk12/1
  cyemi_256/1 -> cfblk13/1
  cfblk6/1 -> cyemi_256/1
  cyemi_257/1 -> cfblk14/1
  cfblk1/1 -> cyemi_257/1
  cyemi_258/1 -> cfblk17/1
  cyemi_259/1 -> cfblk18/1
  cfblk8/1 -> cyemi_259/1
  cyemi_260/1 -> cfblk3/1
  cfblk17/1 -> cyemi_260/1
  cyemi_261/1 -> cfblk4/1
  cfblk18/1 -> cyemi_261/1
  cyemi_262/1 -> cfblk4/2
  cfblk5/1 -> cyemi_262/1
  cyemi_263/1 -> cfblk5/1
  cyemi_264/1 -> cfblk6/1
  cfblk15/1 -> cyemi_264/1
  cyemi_265/1 -> cfblk7/1
  cfblk14/1 -> cyemi_265/1
  cyemi_266/1 -> cfblk8/1
  cfblk10/1 -> cyemi_266/1
  cyemi_267/1 -> cfblk9/1
  cfblk4/1 -> cyemi_267/1

== system sampleModel7126_pp_difftest/cfblk252/cfblk16 ==
  cfblk1 : Inport
  cfblk16 : Inport  Port=2
  Action Port : ActionPort  ActionType=else
  cfblk10 : simulink/Discrete/Difference  ICPrevInput=0.0  OutMin=[]  OutMax=[]  OutDataTypeStr=double  OutputDataTypeScalingMode=double  OutDataType=fixdt(1, 16)  OutScaling=2^-10  DoSatur=off
  cfblk11 : DiscreteIntegrator  SampleTime=-1  OutDataTypeStr=double  ICPrevOutput=DiscIntNeverNeededParam  ICPrevScaledInput=DiscIntNeverNeededParam
  cfblk12 : simulink/Discrete/Transfer Fcn Real Zero  ZeroZ=0.75  ICPrevInput=0.0  DoSatur=off
      settings: SourceProductName=Simulink  SourceProductBaseCode=SL
  cfblk13 : Delay
  cfblk14 : Delay  DelayLengthSource=Input port
      settings: InputPortMap=u0,p1
  cfblk15 : DiscreteFilter
  cfblk3 : Delay  DelayLengthSource=Input port
      settings: InputPortMap=u0,p1
  cfblk4 : simulink/Discrete/Tapped Delay  vinit=0.0  samptime=-1  NumDelays=1  DelayOrder=Oldest  includeCurrent=off
  cfblk5 : simulink/Discrete/Transfer Fcn Lead or Lag  PoleZ=0.95  ZeroZ=0.75  ICPrevOutput=0.0  ICPrevInput=0.0  DoSatur=off
      settings: SourceProductName=Simulink  SourceProductBaseCode=SL
  cfblk6 : Delay  ShowEnablePort=on
      settings: InputPortMap=u0,e6
  cfblk7 : DiscreteTransferFcn
  cfblk8 : simulink/Discrete/Transfer Fcn Lead or Lag  PoleZ=0.95  ZeroZ=0.75  ICPrevOutput=0.0  ICPrevInput=0.0  DoSatur=off
      settings: SourceProductName=Simulink  SourceProductBaseCode=SL
  cfblk9 : UnitDelay  SampleTime=-1
  cyemi_{270..285} (16 alike) : DataTypeConversion  OutDataTypeStr=double
  cfblk2 : Outport
  cfblk17 : Outport  Port=2
  wires:
  cfblk8/1 -> cyemi_270/1, cyemi_281/1
  cfblk9/1 -> cfblk2/1
  cfblk13/1 -> cfblk17/1, cyemi_272/1
  cyemi_270/1 -> cfblk10/1
  cyemi_271/1 -> cfblk11/1
  cfblk4/1 -> cyemi_271/1
  cyemi_272/1 -> cfblk12/1
  cyemi_273/1 -> cfblk13/1
  cfblk10/1 -> cyemi_273/1
  cyemi_274/1 -> cfblk14/1
  cfblk15/1 -> cyemi_274/1, cyemi_275/1
  cyemi_275/1 -> cfblk14/2
  cyemi_276/1 -> cfblk15/1
  cfblk5/1 -> cyemi_276/1
  cyemi_277/1 -> cfblk3/1
  cfblk14/1 -> cyemi_277/1
  cyemi_278/1 -> cfblk3/2
  cfblk16/1 -> cyemi_278/1
  cyemi_279/1 -> cfblk4/1
  cfblk3/1 -> cyemi_279/1
  cyemi_280/1 -> cfblk5/1
  cfblk7/1 -> cyemi_280/1
  cyemi_281/1 -> cfblk6/1
  cyemi_282/1 -> cfblk6/2
  cfblk12/1 -> cyemi_282/1
  cyemi_283/1 -> cfblk7/1
  cfblk1/1 -> cyemi_283/1
  cyemi_284/1 -> cfblk8/1
  cfblk11/1 -> cyemi_284/1
  cyemi_285/1 -> cfblk9/1
  cfblk6/1 -> cyemi_285/1

== system sampleModel7126_pp_difftest/cfblk253/cfblk10 ==
  cfblk1 : Inport
  cfblk12 : Inport  Port=2
  cfblk13 : Inport  Port=3
  cfblk14 : Inport  Port=4
  Action Port : ActionPort  ActionType=else
  cfblk10 : DiscreteFilter
  cfblk11 : DiscreteFir
  cfblk3 : simulink/Discrete/Transfer Fcn First Order  PoleZ=0.95  ICPrevOutput=0.0  DoSatur=off
      settings: SourceProductName=Simulink
  cfblk4 : simulink/Discrete/Difference  ICPrevInput=0.0  OutMin=[]  OutMax=[]  OutDataTypeStr=double  OutputDataTypeScalingMode=double  OutDataType=fixdt(1, 16)  OutScaling=2^-10  DoSatur=off
  cfblk5 : DiscreteStateSpace  SampleTime=-1
  cfblk6 : Delay
  cfblk7 : DiscreteZeroPole  Poles=[0 0.5]  Gain=1  SampleTime=-1
  cfblk8 : Delay
  cfblk9 : UnitDelay  SampleTime=-1
  cyemi_{303..311} (9 alike) : DataTypeConversion  OutDataTypeStr=double
  cfblk2 : Outport
  cfblk15 : Outport  Port=2
  wires:
  cfblk3/1 -> cfblk2/1
  cfblk12/1 -> cfblk15/1
  cyemi_303/1 -> cfblk10/1
  cfblk8/1 -> cyemi_303/1
  cyemi_304/1 -> cfblk11/1
  cfblk10/1 -> cyemi_304/1
  cyemi_305/1 -> cfblk3/1
  cfblk7/1 -> cyemi_305/1
  cyemi_306/1 -> cfblk4/1
  cfblk5/1 -> cyemi_306/1
  cyemi_307/1 -> cfblk5/1
  cfblk14/1 -> cyemi_307/1
  cyemi_308/1 -> cfblk6/1
  cfblk1/1 -> cyemi_308/1
  cyemi_309/1 -> cfblk7/1
  cfblk11/1 -> cyemi_309/1
  cyemi_310/1 -> cfblk8/1
  cfblk13/1 -> cyemi_310/1
  cyemi_311/1 -> cfblk9/1
  cfblk4/1 -> cyemi_311/1

== system sampleModel7126_pp_difftest/cfblk253/cfblk9 ==
  cfblk1 : Inport
  cfblk4 : Inport  Port=2
  cfblk5 : Inport  Port=3
  cfblk6 : Inport  Port=4
  Action Port : ActionPort  ActionType=then
  cfblk3 : DiscreteZeroPole  Poles=[0 0.5]  Gain=1  SampleTime=-1
  cyemi_327 : DataTypeConversion  OutDataTypeStr=double
  cfblk2 : Outport
  cfblk7 : Outport  Port=2
  cfblk8 : Outport  Port=3
  cfblk9 : Outport  Port=4
  wires:
  cfblk1/1 -> cfblk2/1
  cfblk6/1 -> cfblk8/1
  cfblk5/1 -> cfblk7/1
  cfblk3/1 -> cfblk9/1
  cyemi_327/1 -> cfblk3/1
  cfblk4/1 -> cyemi_327/1

== system sampleModel7126_pp_difftest/cfblk256/cfblk11 ==
  cfblk1 : Inport
  cfblk9 : Inport  Port=2
  cfblk10 : Inport  Port=3
  Action Port : ActionPort  ActionType=then
  cfblk3 : simulink/Discrete/Tapped Delay  vinit=0.0  samptime=-1  NumDelays=1  DelayOrder=Oldest  includeCurrent=off
  cfblk4 : simulink/Discrete/Transfer Fcn Real Zero  ZeroZ=0.75  ICPrevInput=0.0  DoSatur=off
      settings: SourceProductName=Simulink  SourceProductBaseCode=SL
  cfblk5 : DiscreteStateSpace  SampleTime=-1
  cfblk6 : DiscreteTransferFcn
  cfblk7 : simulink/Continuous/PID Controller  Controller=PID  TimeDomain=Discrete-time  SampleTime=-1  IntegratorMethod=Forward Euler  FilterMethod=Forward Euler  Form=Parallel  UseFilter=on  ControllerParametersSource=internal  P=1  I=1  D=0  N=100  InitialConditionSource=internal  InitialConditionForIntegrator=0  InitialConditionForFilter=0  ExternalReset=none  LimitOutput=off  UpperSaturationLimit=inf  LowerSaturationLimit=-inf  LinearizeAsGain=off  AntiWindupMode=none  Kb=1  TrackingMode=off  Kt=1  PParamMin=[]  PParamMax=[]  IParamMin=[]  IParamMax=[]  DParamMin=[]  DParamMax=[]  NParamMin=[]  NParamMax=[]  KbParamMin=[]  KbParamMax=[]  KtParamMin=[]  KtParamMax=[]  POutMin=[]  POutMax=[]  IOutMin=[]  IOutMax=[]  DOutMin=[]  DOutMax=[]  NOutMin=[]  NOutMax=[]  KbOutMin=[]  KbOutMax=[]  KtOutMin=[]  KtOutMax=[]  IntegratorOutMin=[]  IntegratorOutMax=[]  FilterOutMin=[]  FilterOutMax=[]  SumOutMin=[]  SumOutMax=[]  SumI1OutMin=[]  SumI1OutMax=[]  SumI2OutMin=[]  SumI2OutMax=[]  SumI3OutMin=[]  SumI3OutMax=[]  SumDOutMin=[]  SumDOutMax=[]  SaturationOutMin=[]  SaturationOutMax=[]  IntegratorContinuousStateAttributes=''  IntegratorStateMustResolveToSignalObject=off  IntegratorRTWStateStorageClass=Auto  FilterContinuousStateAttributes=''  FilterStateMustResolveToSignalObject=off  FilterRTWStateStorageClass=Auto  DifferentiatorICPrevScaledInput=0  DifferentiatorOutMin=[]  DifferentiatorOutMax=[]  FilterDiffOutCoefMin=[]  FilterDiffOutCoefMax=[]  SumDenOutMin=[]  SumDenOutMax=[]  SumNumOutMin=[]  SumNumOutMax=[]  ReciprocalOutMin=[]  ReciprocalOutMax=[]  DivideOutMin=[]  DivideOutMax=[]  TunerSelectOption=Transfer Function Based (PID Tuner App)
  cfblk8 : DiscreteFir
  cyemi_{362..367} (6 alike) : DataTypeConversion  OutDataTypeStr=double
  cfblk2 : Outport
  cfblk11 : Outport  Port=2
  wires:
  cfblk7/1 -> cfblk2/1
  cfblk6/1 -> cfblk11/1
  cyemi_362/1 -> cfblk3/1
  cfblk9/1 -> cyemi_362/1
  cyemi_363/1 -> cfblk4/1
  cfblk1/1 -> cyemi_363/1
  cyemi_364/1 -> cfblk5/1
  cfblk8/1 -> cyemi_364/1
  cyemi_365/1 -> cfblk6/1
  cfblk4/1 -> cyemi_365/1
  cyemi_366/1 -> cfblk7/1
  cfblk5/1 -> cyemi_366/1
  cyemi_367/1 -> cfblk8/1
  cfblk3/1 -> cyemi_367/1

== system sampleModel7126_pp_difftest/cfblk256/cfblk12 ==
  cfblk1 : Inport
  Action Port : ActionPort  ActionType=else
  cfblk3 : DiscreteTransferFcn
  cfblk4 : simulink/Discrete/Difference  ICPrevInput=0.0  OutMin=[]  OutMax=[]  OutDataTypeStr=double  OutputDataTypeScalingMode=double  OutDataType=fixdt(1, 16)  OutScaling=2^-10  DoSatur=off
  cfblk5 : DiscreteIntegrator  SampleTime=-1  OutDataTypeStr=double  ICPrevOutput=DiscIntNeverNeededParam  ICPrevScaledInput=DiscIntNeverNeededParam
  cfblk6 : Delay
  cyemi_{369..372} (4 alike) : DataTypeConversion  OutDataTypeStr=double
  cfblk2 : Outport
  cfblk7 : Outport  Port=2
  cfblk8 : Outport  Port=3
  wires:
  cfblk4/1 -> cfblk7/1, cfblk2/1
  cfblk3/1 -> cfblk8/1, cyemi_371/1
  cyemi_369/1 -> cfblk3/1
  cfblk1/1 -> cyemi_369/1
  cyemi_370/1 -> cfblk4/1
  cfblk6/1 -> cyemi_370/1
  cyemi_371/1 -> cfblk5/1
  cyemi_372/1 -> cfblk6/1
  cfblk5/1 -> cyemi_372/1

== system sampleModel7126_pp_difftest/cfblk259/cfblk10 ==
  cfblk1 : Inport
  cfblk10 : Inport  Port=2
  cfblk11 : Inport  Port=3
  cfblk12 : Inport  Port=4
  Action Port : ActionPort  ActionType=else
  cfblk13 : Delay
  cfblk3 : DiscreteZeroPole  Poles=[0 0.5]  Gain=1  SampleTime=-1
  cfblk4 : Delay  ShowEnablePort=on
      settings: InputPortMap=u0,e6
  cfblk5 : DiscreteStateSpace  SampleTime=-1
  cfblk6 : DiscreteTransferFcn
  cfblk7 : DiscreteStateSpace  SampleTime=-1
  cfblk8 : simulink/Discrete/Transfer Fcn First Order  PoleZ=0.95  ICPrevOutput=0.0  DoSatur=off
      settings: SourceProductName=Simulink
  cfblk9 : DiscreteTransferFcn
  cyemi_{412..420} (9 alike) : DataTypeConversion  OutDataTypeStr=double
  cfblk2 : Outport
  wires:
  cfblk10/1 -> cfblk2/1
  cyemi_412/1 -> cfblk13/1
  cfblk6/1 -> cyemi_412/1
  cyemi_413/1 -> cfblk3/1
  cfblk5/1 -> cyemi_413/1
  cyemi_414/1 -> cfblk4/1
  cfblk12/1 -> cyemi_414/1
  cyemi_415/1 -> cfblk4/2
  cfblk13/1 -> cyemi_415/1
  cyemi_416/1 -> cfblk5/1
  cfblk11/1 -> cyemi_416/1
  cyemi_417/1 -> cfblk6/1
  cfblk4/1 -> cyemi_417/1
  cyemi_418/1 -> cfblk7/1
  cfblk9/1 -> cyemi_418/1
  cyemi_419/1 -> cfblk8/1
  cfblk3/1 -> cyemi_419/1
  cyemi_420/1 -> cfblk9/1
  cfblk1/1 -> cyemi_420/1

== system sampleModel7126_pp_difftest/cfblk259/cfblk9 ==
  cfblk1 : Inport
  cfblk11 : Inport  Port=2
  Action Port : ActionPort  ActionType=then
  cfblk10 : simulink/Discrete/Difference  ICPrevInput=0.0  OutMin=[]  OutMax=[]  OutDataTypeStr=double  OutputDataTypeScalingMode=double  OutDataType=fixdt(1, 16)  OutScaling=2^-10  DoSatur=off
  cfblk14 : Delay
  cfblk15 : Delay
  cfblk3 : simulink/Discrete/Tapped Delay  vinit=0.0  samptime=-1  NumDelays=1  DelayOrder=Oldest  includeCurrent=off
  cfblk4 : Delay  ShowEnablePort=on
      settings: InputPortMap=u0,e6
  cfblk5 : simulink/Discrete/Transfer Fcn First Order  PoleZ=0.95  ICPrevOutput=0.0  DoSatur=off
      settings: SourceProductName=Simulink
  cfblk6 : DiscreteFilter
  cfblk7 : Delay  DelayLengthSource=Input port
      settings: InputPortMap=u0,p1
  cfblk8 : Delay  DelayLengthSource=Input port
      settings: InputPortMap=u0,p1
  cfblk9 : Delay  DelayLengthSource=Input port
      settings: InputPortMap=u0,p1
  cyemi_{432..445} (14 alike) : DataTypeConversion  OutDataTypeStr=double
  cfblk2 : Outport
  cfblk12 : Outport  Port=2
  cfblk13 : Outport  Port=3
  wires:
  cfblk6/1 -> cyemi_434/1, cyemi_438/1
  cfblk8/1 -> cfblk12/1, cfblk13/1, cyemi_432/1
  cfblk3/1 -> cfblk2/1, cyemi_439/1
  cfblk10/1 -> cyemi_435/1, cyemi_441/1
  cyemi_432/1 -> cfblk10/1
  cyemi_433/1 -> cfblk14/1
  cfblk7/1 -> cyemi_433/1
  cyemi_434/1 -> cfblk15/1
  cyemi_435/1 -> cfblk3/1
  cyemi_436/1 -> cfblk4/1
  cfblk14/1 -> cyemi_436/1
  cyemi_437/1 -> cfblk4/2
  cfblk9/1 -> cyemi_437/1
  cyemi_438/1 -> cfblk5/1
  cyemi_439/1 -> cfblk6/1
  cyemi_440/1 -> cfblk7/1
  cfblk5/1 -> cyemi_440/1
  cyemi_441/1 -> cfblk7/2
  cyemi_442/1 -> cfblk8/1
  cfblk4/1 -> cyemi_442/1
  cyemi_443/1 -> cfblk8/2
  cfblk15/1 -> cyemi_443/1
  cyemi_444/1 -> cfblk9/1
  cfblk11/1 -> cyemi_444/1
  cyemi_445/1 -> cfblk9/2
  cfblk1/1 -> cyemi_445/1
